simulink model "cart_pend_DMDc"  (R2019b)
settings: Solver=FixedStepAuto  StartTime=0.0  StopTime=200  FixedStep=0.01  RelTol=1e-3
values from neighbouring files (symbols this model uses):
  A = [0.969169519504925  -0.246386829627017;  0.049277365925403  0.993808202467626]    [DMDc_MW.m]    (also in DMDc_param_sweep.m = real(A); EKF_msd_estimator.m = [0, 1; -k/m, -b/m]; HAVOK.m = AB(:,1:q*m); HAVOK_param_sweep.m = real(A))
  B = [0.049277365925403; 0.001238359506475]    [DMDc_MW.m]    (also in DMDc_param_sweep.m = AB(:,(q*m+1):end); EKF_estimator.m = zeros(nx,1); EKF_msd_estimator.m = [0; 1/m]; HAVOK.m = AB(:,(q*m+1):end))
settings Model: PacingRate=3  Creator=Murray  LastModifiedBy=Murray
settings SolverCC: AlgebraicLoopSolver=LineSearch
settings DebuggingCC: UnderSpecifiedDimensionMsg=warning

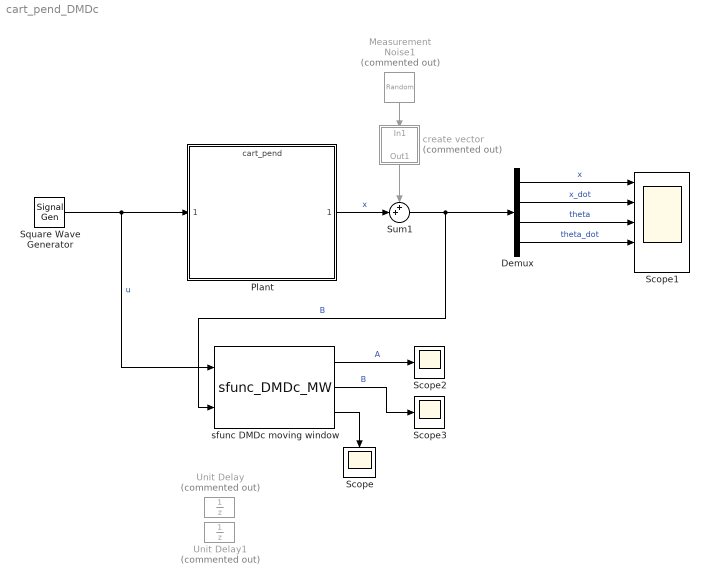
== system cart_pend_DMDc ==
  Demux : Demux
  Measurement Noise1 : RandomNumber  Commented=on  Variance=0.001  SampleTime=0.05
  Plant : ModelReference  ModelNameDialog=cart_pend  SimulationMode=Normal  ModelReferenceVersion=1.16
  Scope : Scope
  Scope1 : Scope  NumInputPorts=5
  Scope2 : Scope
  Scope3 : Scope
  Square Wave Generator : SignalGenerator  WaveForm=square  Amplitude=5  Frequency=1/10
  Sum1 : Sum  Inputs=++|
  Unit Delay : UnitDelay  Commented=on  InitialCondition=A  SampleTime=0.2  HasFrameUpgradeWarning=on
  Unit Delay1 : UnitDelay  Commented=on  InitialCondition=B  SampleTime=0.2  HasFrameUpgradeWarning=on
  create vector : Subsystem  Commented=on
  sfunc DMDc moving window : M-S-Function  FunctionName=sfunc_DMDc_MW  Parameters=mpc1.Ts, 500, 4, 1
      mask Display:
      | port_label('input', 1, 'u')
      | port_label('input', 2, 'x')
      | 
      | port_label('output', 1, 'A')
      | port_label('output', 2, 'B')
      | port_label('output', 3, 'MSE')
  wires:
  sfunc DMDc moving window/1 -> Scope2/1  "A"
  sfunc DMDc moving window/2 -> Scope3/1  "B"
  sfunc DMDc moving window/3 -> Scope/1
  Square Wave Generator/1 -> sfunc DMDc moving window/1, Plant/1  "u"
  Demux/1 -> Scope1/1  "x"
  Demux/2 -> Scope1/2  "x_dot"
  Demux/3 -> Scope1/3  "theta"
  Demux/4 -> Scope1/4  "theta_dot"
  Measurement Noise1/1 -> create vector/1(In1)
  create vector/1(Out1) -> Sum1/1
  Plant/1 -> Sum1/2  "x"
  Sum1/1 -> sfunc DMDc moving window/2, Demux/1  "B"

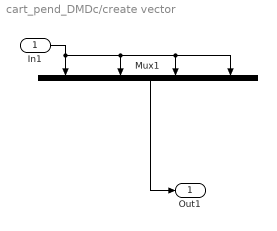
== system cart_pend_DMDc/create vector ==
  In1 : Inport
  Mux1 : Mux
  Out1 : Outport
  wires:
  In1/1 -> Mux1/4, Mux1/3, Mux1/2, Mux1/1
  Mux1/1 -> Out1/1
